simulink model "ex8"  (R2015a)
settings: Solver=ode3  StartTime=0.0  StopTime=30  FixedStep=0.01  RelTol=1e-3
undefined symbols (not defined in the file): l
libraries: simulink x1
settings Model: Creator=fschalle  LastModifiedBy=fschalle

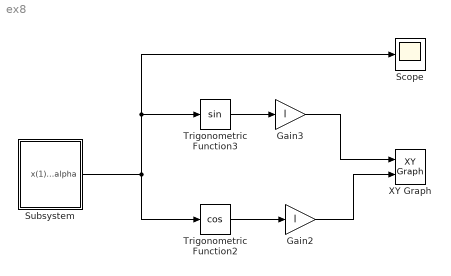
== system ex8 ==
  Gain2 : Gain  Gain=l
  Gain3 : Gain  Gain=l
  Scope : Scope
      settings: YMin=-7  YMax=7
  Subsystem : Subsystem
  Trigonometric Function2 : Trigonometry  Operator=cos
  Trigonometric Function3 : Trigonometry
  XY Graph : simulink/Sinks/XY Graph  xmin=-1  xmax=1  ymin=-1  ymax=1  st=-1
  wires:
  Trigonometric Function2/1 -> Gain2/1
  Trigonometric Function3/1 -> Gain3/1
  Gain2/1 -> XY Graph/2
  Gain3/1 -> XY Graph/1
  Subsystem/1(x(1)=alpha) -> Trigonometric Function2/1, Scope/1, Trigonometric Function3/1

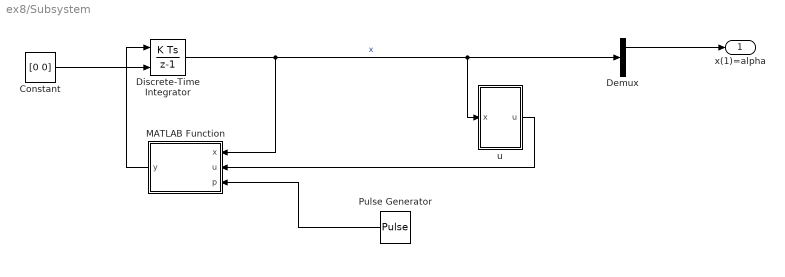
== system ex8/Subsystem ==
  Constant : Constant  Value=[0 0]
  Demux : Demux  Outputs=2
  Discrete-Time Integrator : DiscreteIntegrator  InitialConditionSource=external  InitialConditionSetting=State (most efficient)  SampleTime=0.01
  MATLAB Function : MATLAB Function  TreatAsAtomicUnit=on
  Pulse Generator : DiscretePulseGenerator  PulseType=Time based  Amplitude=0.1  Period=1  PulseWidth=20
  "u " : Subsystem
  x(1)=alpha : Outport
  wires:
  Constant/1 -> Discrete-Time Integrator/2
  Discrete-Time Integrator/1 -> MATLAB Function/1(x), Demux/1, "u "/1(x)  "x"
  MATLAB Function/1(y) -> Discrete-Time Integrator/1
  Demux/1 -> x(1)=alpha/1
  "u "/1(u) -> MATLAB Function/2(u)
  Pulse Generator/1 -> MATLAB Function/3(p)

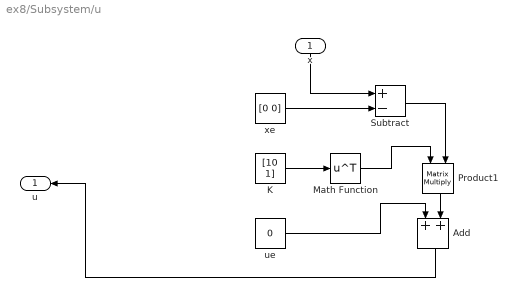
== system ex8/Subsystem/u  ==
  x : Inport
  Add : Sum
  "K " : Constant  Value=[10 1]
  Math Function : Math  Operator=transpose  SaturateOnIntegerOverflow=on
  Product1 : Product  Multiplication=Matrix(*)
  Subtract : Sum  Inputs=+-
  ue : Constant  Value=0
  xe : Constant  Value=[0 0]
  u : Outport
  wires:
  Add/1 -> u/1
  x/1 -> Subtract/1
  xe/1 -> Subtract/2
  ue/1 -> Add/1
  Product1/1 -> Add/2
  Subtract/1 -> Product1/2
  "K "/1 -> Math Function/1
  Math Function/1 -> Product1/1

== matlab function ex8/Subsystem/MATLAB Function ==
  data: x input; u input; y output; p input
function y = fcn(x,u,p)
%#codegen
g=9.81;
l=1;
y = [x(2)+p ; (g/l*sin(x(1))-1/l*u*cos(x(1)))];
